simulink model "dip_ekf_sim_discrete_student"  (R2022b)
settings: Solver=ode4  StartTime=0.0  StopTime=10  FixedStep=timeStep  MaxStep=0.05  RelTol=1e-3  EnableMultiTasking=on
values from neighbouring files (symbols this model uses):
  hx0e = [hx0';P0(:)]    [dip_sim_ekf_ini.m]
  par = [l1,l2,l_S1,l_S2,m_G1,m_G2,J_G1xx,J_G2xx,k_G1,k_G2,g]    [dip_sim_ekf_ini.m]
  Q = eye(6)*0.00001    [dip_sim_ekf_ini.m]
  R = eye(3)*0.001    [dip_sim_ekf_ini.m]
settings Model: Creator=ut  LastModifiedBy=15043
settings SolverCC: AlgebraicLoopSolver=TrustRegion
settings DataIOCC: LimitDataPoints=on  SaveFormat=Array  SignalLoggingSaveFormat=ModelDataLogs  ReturnWorkspaceOutputs=off
settings OptimizationCC: ExpressionDepthLimit=2147483647  InitFltsAndDblsToZero=on  LifeSpan=inf
settings DebuggingCC: SaveWithParameterizedLinksMsg=none  UnderspecifiedInitializationDetection=Classic  MergeDetectMultiDrivingBlocksExec=none  SignalResolutionControl=TryResolveAllWithWarning  SolverPrmCheckMsg=warning  MultiTaskDSMMsg=warning  MultiTaskCondExecSysMsg=none  FcnCallInpInsideContextMsg=warning  UnconnectedInputMsg=warning  UnconnectedOutputMsg=warning  UnconnectedLineMsg=warning  StateNameClashWarn=warning  SFUnexpectedBacktrackingDiag=warning  SFNoUnconditionalDefaultTransitionDiag=warning  SFExecutionAtInitializationDiag=none  SFMachineParentedDataDiag=warning  ArithmeticOperatorsInVariantConditions=warning
settings HardwareCC: ProdBitPerPointer=32  ProdBitPerSizeT=32  ProdBitPerPtrDiffT=32  ProdLargestAtomicFloat=None  ProdIntDivRoundTo=Undefined  ProdEndianess=Unspecified  ProdWordSize=32  ProdHWDeviceType=32-bit Generic
settings ModelReferenceCC: EnableRefExpFcnMdlSchedulingChecks=on  PropagateSignalLabelsOutOfModel=off
settings SFSimCC: SimUseLocalCustomCode=off  CustomCodeUndefinedFunction=UseInterfaceOnly
settings RTWCC: RTWUseLocalCustomCode=off
settings CodeAppCC: StateflowObjectComments=on
settings GRTTargetCC: TargetFcnLib=ansi_tfl_tmw.mat  TargetLangStandard=C89/C90 (ANSI)  CombineOutputUpdateFcns=off  GRTInterface=on
settings ConfigComp: CovMetricSettings=dw  CovSaveCumulativeToWorkspaceVar=on  CovSaveSingleToWorkspaceVar=on  CovExternalEMLEnable=off

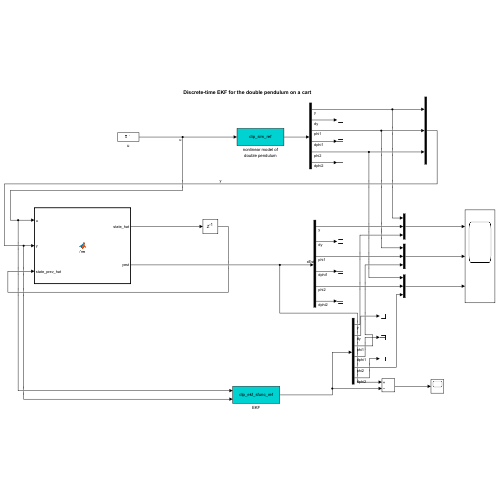
[thumbnail: Simulink's stored preview of the top-level diagram]
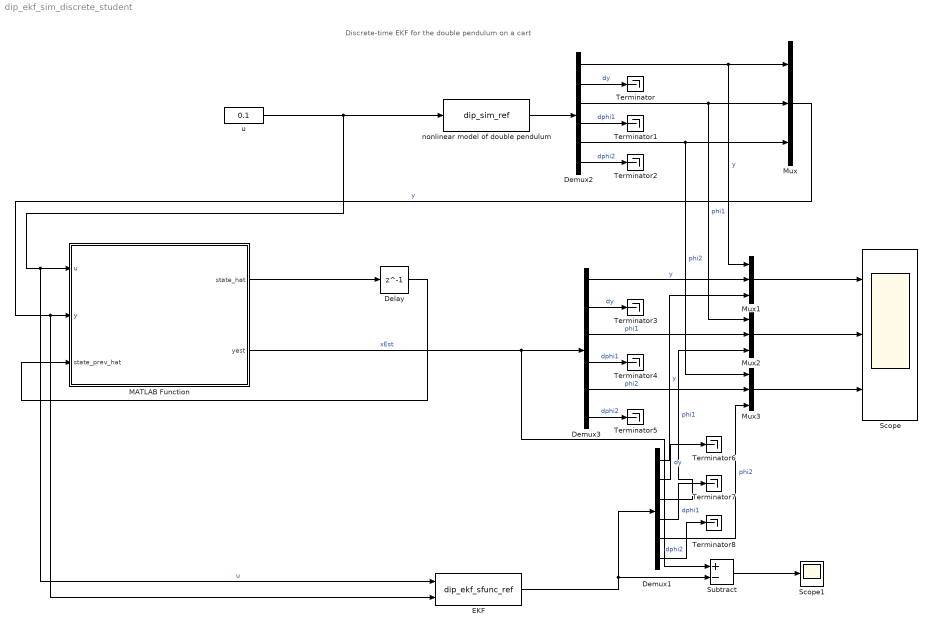
== system dip_ekf_sim_discrete_student ==
  note: Discrete-time EKF for the double pendulum on a cart
  Delay : Delay  DelayLength=1  InitialCondition=hx0e
  Demux1 : Demux  Outputs=6
  Demux2 : Demux  Outputs=6
  Demux3 : Demux  Outputs=6
  EKF : M-S-Function  FunctionName=dip_ekf_sfunc_ref  Parameters=hx0e,Q,R
  MATLAB Function : MATLAB Function  TreatAsAtomicUnit=on
  Mux{,1..3} (4 alike) : Mux  Inputs=3
  Scope : Scope  NumInputPorts=3
  Scope1 : Scope
  Subtract : Sum  Inputs=+-
  Terminator{,1..8} (9 alike) : Terminator
  nonlinear model of double pendulum : M-S-Function  FunctionName=dip_sim_ref  Parameters=x0
  u : Constant  Value=0.1
  wires:
  u/1 -> nonlinear model of double pendulum/1, EKF/1, MATLAB Function/1(u)  "u"
  Demux2/1 -> Mux1/1, Mux/1  "y"
  Demux2/3 -> Mux2/1, Mux/2  "phi1"
  Demux2/5 -> Mux3/1, Mux/3  "phi2"
  Demux2/2 -> Terminator/1  "dy"
  Demux2/4 -> Terminator1/1  "dphi1"
  Demux2/6 -> Terminator2/1  "dphi2"
  Demux3/5 -> Mux3/2  "phi2"
  Demux3/2 -> Terminator3/1  "dy"
  Demux3/3 -> Mux2/2  "phi1"
  Demux3/4 -> Terminator4/1  "dphi1"
  Demux3/6 -> Terminator5/1  "dphi2"
  Demux3/1 -> Mux1/2  "y"
  Mux1/1 -> Scope/1
  Mux2/1 -> Scope/2
  Mux3/1 -> Scope/3
  Subtract/1 -> Scope1/1
  Mux/1 -> EKF/2, MATLAB Function/2(y)  "y"
  nonlinear model of double pendulum/1 -> Demux2/1
  Demux1/6 -> Terminator8/1  "dphi2"
  Demux1/2 -> Terminator6/1  "dy"
  Demux1/4 -> Terminator7/1  "dphi1"
  Demux1/5 -> Mux3/3  "phi2"
  Demux1/3 -> Mux2/3  "phi1"
  Demux1/1 -> Mux1/3  "y"
  EKF/1 -> Subtract/2, Demux1/1
  MATLAB Function/2(yest) -> Subtract/1, Demux3/1  "xEst"
  MATLAB Function/1(state_hat) -> Delay/1
  Delay/1 -> MATLAB Function/3(state_prev_hat)

== matlab function dip_ekf_sim_discrete_student/MATLAB Function ==
  data: u input; state_hat output; y input; state_prev_hat input; R parameter; Q parameter; par parameter; yest output
function [state_hat, yest] = fcn(u, y, state_prev_hat, R, Q, par)
    h = @(x) [x(1); x(3); x(5)];
    H = [1 0 0 0 0 0; 0 0 1 0 0 0; 0 0 0 0 1 0;];
    timeStep = 0.01;
    x_hat = state_prev_hat(1:6, :);
    P = reshape( state_prev_hat(7:end), 6,6);
    
    %F = Fjac( x_hat, u, par);
    s1 = f(x_hat, u, par);
    s2 = f(x_hat+timeStep/2*s1, u, par);
    s3 = f(x_hat+timeStep/2*s2, u, par);
    s4 = f(x_hat+timeStep*s3, u, par);
    S1 = Fjac( x_hat, u, par);
    S2 = Fjac( x_hat + timeStep/2*s1, u, par)*(eye(6) + (timeStep/2)*S1 );
    S3 = Fjac( x_hat + timeStep/2*s2, u, par)*(eye(6) + (timeStep/2)*S2 );
    S4 = Fjac( x_hat + timeStep*s3, u, par)*(eye(6) + timeStep*S3 );
    F = eye(6) + (timeStep/6)*( S1 + 2*S2 + 2*S3 + S4 );
    fd = x_hat + (timeStep/6)*( s1 + 2*s2 + 2*s3 + s4 );
    
    x_hatm = fd;
    Pm = F*P*F' + Q;

    K = Pm*H'*inv((H*Pm*H'+ R));
    %L = P*(H')/R;
    
    x_hat = x_hatm + K*(y-h(x_hatm));
    P = ( eye(6) - K*H)*Pm ;
    
     
    state_hat = [x_hat; P(:);];
    yest = x_hat;
end




function [dx, y] = f(x,a_w,par)
%YEVY
%    EXPR = YEVY(T,IN2,PARAM76,PARAM77,PARAM78,PARAM79,PARAM80,PARAM81,PARAM82,PARAM83,PARAM84,PARAM85,PARAM86,PARAM87)

%    This function was generated by the Symbolic Math Toolbox version 9.2.
%    21-Nov-2022 21:11:29

l1 = par(1);
l2 = par(2);
l_S1 = par(3);
l_S2 = par(4);
m_G1 = par(5);
m_G2 = par(6);
J_G1xx = par(7);
J_G2xx = par(8);
k_G1 = par(9);
k_G2 = par(10);
g = par(11);



%Version: 1.1
Dphi1t = x(4,:);
Dphi2t = x(6,:);
Dyt = x(2,:);
phi1 = x(3,:);
phi2 = x(5,:);
t2 = cos(phi1);
t3 = cos(phi2);
t4 = sin(phi1);
t5 = sin(phi2);
t6 = J_G1xx.*J_G2xx;
t7 = Dphi1t.^2;
t8 = Dphi2t.^2;
t9 = m_G2.^2;
t10 = l_S1.^2;
t11 = l_S2.^2;
t12 = l1.^2;
t13 = -phi2;
t14 = m_G1.*J_G2xx.*t10;
t15 = m_G2.*J_G1xx.*t11;
t16 = m_G2.*J_G2xx.*t12;
t17 = phi1+t13;
t21 = m_G1.*m_G2.*t10.*t11;
t22 = t9.*t11.*t12;
t18 = cos(t17);
t19 = sin(t17);
t20 = t18.^2;
t23 = Dphi1t.*m_G2.*k_G2.*l_S2.*l1.*t18;
t24 = Dphi2t.*m_G2.*k_G2.*l_S2.*l1.*t18;
t25 = -t24;
t26 = t20.*t22;
t27 = -t26;
t28 = t6+t14+t15+t16+t21+t22+t27;
t29 = 1.0./t28;
mt1 = [Dyt;a_w;Dphi1t;-t29.*(t23+t25+Dphi1t.*k_G1.*J_G2xx+Dphi1t.*k_G2.*J_G2xx-Dphi2t.*k_G2.*J_G2xx+t7.*t18.*t19.*t22+Dphi1t.*m_G2.*k_G1.*t11+Dphi1t.*m_G2.*k_G2.*t11-Dphi2t.*m_G2.*k_G2.*t11+a_w.*m_G1.*J_G2xx.*l_S1.*t2+a_w.*m_G2.*J_G2xx.*l1.*t2-g.*m_G1.*J_G2xx.*l_S1.*t4-g.*m_G2.*J_G2xx.*l1.*t4+a_w.*l1.*t2.*t9.*t11-g.*l1.*t4.*t9.*t11+l_S2.^3.*l1.*t8.*t9.*t19+a_w.*m_G1.*m_G2.*l_S1.*t2.*t11-g.*m_G1.*m_G2.*l_S1.*t4.*t11+m_G2.*J_G2xx.*l_S2.*l1.*t8.*t19-a_w.*l1.*t3.*t9.*t11.*t18+g.*l1.*t5.*t9.*t11.*t18);Dphi2t];
mt2 = [t29.*(t23+t25+Dphi1t.*k_G2.*J_G1xx-Dphi2t.*k_G2.*J_G1xx+t8.*t18.*t19.*t22+Dphi1t.*m_G1.*k_G2.*t10-Dphi2t.*m_G1.*k_G2.*t10+Dphi1t.*m_G2.*k_G2.*t12-Dphi2t.*m_G2.*k_G2.*t12-a_w.*m_G2.*J_G1xx.*l_S2.*t3+g.*m_G2.*J_G1xx.*l_S2.*t5-a_w.*l_S2.*t3.*t9.*t12+g.*l_S2.*t5.*t9.*t12+l_S2.*l1.^3.*t7.*t9.*t19-a_w.*m_G1.*m_G2.*l_S2.*t3.*t10+g.*m_G1.*m_G2.*l_S2.*t5.*t10+m_G2.*J_G1xx.*l_S2.*l1.*t7.*t19+a_w.*l_S2.*t2.*t9.*t12.*t18-g.*l_S2.*t4.*t9.*t12.*t18+Dphi1t.*m_G2.*k_G1.*l_S2.*l1.*t18+m_G1.*m_G2.*l_S2.*l1.*t7.*t10.*t19+a_w.*m_G1.*m_G2.*l_S1.*l_S2.*l1.*t2.*t18-g.*m_G1.*m_G2.*l_S1.*l_S2.*l1.*t4.*t18)];

dx = [mt1;mt2];
y = x;
end

 



function df = Fjac( x, a_w, par )
%FJACSYM
%    DF = FJACSYM(J_G1XX,J_G2XX,A_W,DPHI1_T,DPHI2_T,G,K_G1,K_G2,L1,L_S1,L_S2,M_G1,M_G2,PHI1_T,PHI2_T)

%    This function was generated by the Symbolic Math Toolbox version 8.0.
%    21-Nov-2022 22:25:07
phi1_t = x(3);
phi2_t = x(5);
dphi1_t = x(4);
dphi2_t = x(6);


l1 = par(1);
l2 = par(2);
l_S1 = par(3);
l_S2 = par(4);
m_G1 = par(5);
m_G2 = par(6);
J_G1xx = par(7);
J_G2xx = par(8);
k_G1 = par(9);
k_G2 = par(10);
g = par(11);




%Version: 1.1
t2 = l1.^2;
t3 = l_S2.^2;
t4 = m_G2.^2;
t7 = phi1_t-phi2_t;
t5 = cos(t7);
t6 = l_S1.^2;
t8 = cos(phi1_t);
t9 = sin(phi1_t);
t10 = t5.^2;
t11 = dphi1_t.^2;
t12 = sin(t7);
t13 = dphi2_t.^2;
t14 = J_G1xx.*J_G2xx;
t15 = t2.*t3.*t4;
t16 = J_G2xx.*m_G2.*t2;
t17 = J_G2xx.*m_G1.*t6;
t18 = J_G1xx.*m_G2.*t3;
t19 = m_G1.*m_G2.*t3.*t6;
t23 = t2.*t3.*t4.*t10;
t20 = t14+t15+t16+t17+t18+t19-t23;
t21 = cos(phi2_t);
t22 = sin(phi2_t);
t24 = 1.0./t20;
t25 = t12.^2;
t26 = t2.*t3.*t4.*t11.*t25;
t27 = dphi1_t.*k_G2.*l1.*l_S2.*m_G2.*t12;
t28 = g.*l1.*t3.*t4.*t12.*t22;
t29 = 1.0./t20.^2;
t30 = J_G2xx.*dphi1_t.*k_G1;
t31 = J_G2xx.*dphi1_t.*k_G2;
t32 = dphi1_t.*k_G1.*m_G2.*t3;
t33 = dphi1_t.*k_G2.*m_G2.*t3;
t34 = l1.*l_S2.*t3.*t4.*t12.*t13;
t35 = a_w.*l1.*t3.*t4.*t8;
t36 = J_G2xx.*a_w.*l1.*m_G2.*t8;
t37 = J_G2xx.*a_w.*l_S1.*m_G1.*t8;
t38 = dphi1_t.*k_G2.*l1.*l_S2.*m_G2.*t5;
t39 = t2.*t3.*t4.*t5.*t11.*t12;
t40 = a_w.*l_S1.*m_G1.*m_G2.*t3.*t8;
t41 = g.*l1.*t3.*t4.*t5.*t22;
t42 = J_G2xx.*l1.*l_S2.*m_G2.*t12.*t13;
t48 = dphi2_t.*k_G2.*l1.*l_S2.*m_G2.*t5;
t43 = t30+t31+t32+t33+t34+t35+t36+t37+t38+t39+t40+t41+t42-t48-J_G2xx.*dphi2_t.*k_G2-dphi2_t.*k_G2.*m_G2.*t3-J_G2xx.*g.*l1.*m_G2.*t9-J_G2xx.*g.*l_S1.*m_G1.*t9-g.*l1.*t3.*t4.*t9-g.*l_S1.*m_G1.*m_G2.*t3.*t9-a_w.*l1.*t3.*t4.*t5.*t21;
t44 = t2.*t3.*t4.*t5.*t12.*t29.*t43.*2.0;
t45 = J_G2xx.*k_G2;
t46 = k_G2.*m_G2.*t3;
t47 = k_G2.*l1.*l_S2.*m_G2.*t5;
t49 = t2.*t3.*t4.*t13.*t25;
t50 = dphi1_t.*k_G1.*l1.*l_S2.*m_G2.*t12;
t51 = a_w.*l_S2.*t2.*t4.*t8.*t12;
t52 = a_w.*l1.*l_S1.*l_S2.*m_G1.*m_G2.*t8.*t12;
t53 = J_G1xx.*dphi1_t.*k_G2;
t54 = dphi1_t.*k_G2.*m_G2.*t2;
t55 = dphi1_t.*k_G2.*m_G1.*t6;
t56 = l1.*l_S2.*t2.*t4.*t11.*t12;
t57 = g.*l_S2.*t2.*t4.*t22;
t58 = J_G1xx.*g.*l_S2.*m_G2.*t22;
t59 = dphi1_t.*k_G1.*l1.*l_S2.*m_G2.*t5;
t60 = a_w.*l_S2.*t2.*t4.*t5.*t8;
t61 = t2.*t3.*t4.*t5.*t12.*t13;
t62 = g.*l_S2.*m_G1.*m_G2.*t6.*t22;
t63 = J_G1xx.*l1.*l_S2.*m_G2.*t11.*t12;
t64 = l1.*l_S2.*m_G1.*m_G2.*t6.*t11.*t12;
t65 = a_w.*l1.*l_S1.*l_S2.*m_G1.*m_G2.*t5.*t8;
t66 = t38-t48+t53+t54+t55+t56+t57+t58+t59+t60+t61+t62+t63+t64+t65-J_G1xx.*dphi2_t.*k_G2-dphi2_t.*k_G2.*m_G2.*t2-dphi2_t.*k_G2.*m_G1.*t6-J_G1xx.*a_w.*l_S2.*m_G2.*t21-a_w.*l_S2.*t2.*t4.*t21-g.*l_S2.*t2.*t4.*t5.*t9-a_w.*l_S2.*m_G1.*m_G2.*t6.*t21-g.*l1.*l_S1.*l_S2.*m_G1.*m_G2.*t5.*t9;
t67 = J_G1xx.*k_G2;
t68 = k_G2.*m_G2.*t2;
t69 = k_G2.*m_G1.*t6;
df = reshape([0.0,0.0,0.0,0.0,0.0,0.0,1.0,0.0,0.0,0.0,0.0,0.0,0.0,0.0,0.0,t44+t24.*(t26+t27+t28+J_G2xx.*a_w.*l1.*m_G2.*t9+J_G2xx.*a_w.*l_S1.*m_G1.*t9+J_G2xx.*g.*l1.*m_G2.*t8+J_G2xx.*g.*l_S1.*m_G1.*t8+a_w.*l1.*t3.*t4.*t9+g.*l1.*t3.*t4.*t8-t2.*t3.*t4.*t10.*t11-l1.*l_S2.*t3.*t4.*t5.*t13-J_G2xx.*l1.*l_S2.*m_G2.*t5.*t13-dphi2_t.*k_G2.*l1.*l_S2.*m_G2.*t12+a_w.*l_S1.*m_G1.*m_G2.*t3.*t9+g.*l_S1.*m_G1.*m_G2.*t3.*t8-a_w.*l1.*t3.*t4.*t12.*t21),0.0,-t24.*(t27+t49+t50+t51+t52-t2.*t3.*t4.*t10.*t13+g.*l_S2.*t2.*t4.*t5.*t8-g.*l_S2.*t2.*t4.*t9.*t12-l1.*l_S2.*t2.*t4.*t5.*t11-J_G1xx.*l1.*l_S2.*m_G2.*t5.*t11-dphi2_t.*k_G2.*l1.*l_S2.*m_G2.*t12+a_w.*l_S2.*t2.*t4.*t5.*t9-l1.*l_S2.*m_G1.*m_G2.*t5.*t6.*t11+a_w.*l1.*l_S1.*l_S2.*m_G1.*m_G2.*t5.*t9+g.*l1.*l_S1.*l_S2.*m_G1.*m_G2.*t5.*t8-g.*l1.*l_S1.*l_S2.*m_G1.*m_G2.*t9.*t12)-t2.*t3.*t4.*t5.*t12.*t29.*t66.*2.0,0.0,0.0,1.0,-t24.*(t45+t46+t47+J_G2xx.*k_G1+k_G1.*m_G2.*t3+dphi1_t.*t2.*t3.*t4.*t5.*t12.*2.0),0.0,t24.*(t47+t67+t68+t69+k_G1.*l1.*l_S2.*m_G2.*t5+J_G1xx.*dphi1_t.*l1.*l_S2.*m_G2.*t12.*2.0+dphi1_t.*l1.*l_S2.*t2.*t4.*t12.*2.0+dphi1_t.*l1.*l_S2.*m_G1.*m_G2.*t6.*t12.*2.0),0.0,0.0,0.0,-t44-t24.*(t26+t27+t28-t2.*t3.*t4.*t10.*t11+g.*l1.*t3.*t4.*t5.*t21-l1.*l_S2.*t3.*t4.*t5.*t13-J_G2xx.*l1.*l_S2.*m_G2.*t5.*t13-dphi2_t.*k_G2.*l1.*l_S2.*m_G2.*t12+a_w.*l1.*t3.*t4.*t5.*t22-a_w.*l1.*t3.*t4.*t12.*t21),0.0,t24.*(t27+t49+t50+t51+t52+J_G1xx.*a_w.*l_S2.*m_G2.*t22+J_G1xx.*g.*l_S2.*m_G2.*t21+a_w.*l_S2.*t2.*t4.*t22+g.*l_S2.*t2.*t4.*t21-t2.*t3.*t4.*t10.*t13-g.*l_S2.*t2.*t4.*t9.*t12-l1.*l_S2.*t2.*t4.*t5.*t11-J_G1xx.*l1.*l_S2.*m_G2.*t5.*t11-dphi2_t.*k_G2.*l1.*l_S2.*m_G2.*t12+a_w.*l_S2.*m_G1.*m_G2.*t6.*t22+g.*l_S2.*m_G1.*m_G2.*t6.*t21-l1.*l_S2.*m_G1.*m_G2.*t5.*t6.*t11-g.*l1.*l_S1.*l_S2.*m_G1.*m_G2.*t9.*t12)+t2.*t3.*t4.*t5.*t12.*t29.*t66.*2.0,0.0,0.0,0.0,t24.*(t45+t46+t47-J_G2xx.*dphi2_t.*l1.*l_S2.*m_G2.*t12.*2.0-dphi2_t.*l1.*l_S2.*t3.*t4.*t12.*2.0),1.0,-t24.*(t47+t67+t68+t69-dphi2_t.*t2.*t3.*t4.*t5.*t12.*2.0)],[6,6]);
end
